simulink model "Model_Architecture"  (R2025b)
settings: Solver=VariableStepAuto  StartTime=0.0  StopTime=10.0  RelTol=1e-3
undefined symbols (not defined in the file): Selector
settings Model: Creator=dehc5901  LastModifiedBy=dehc5901

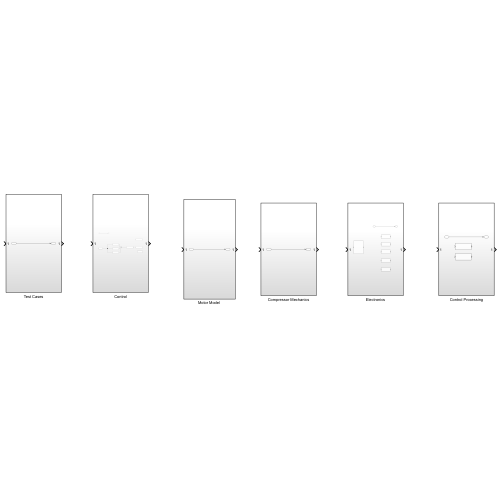
[thumbnail: Simulink's stored preview of the top-level diagram]
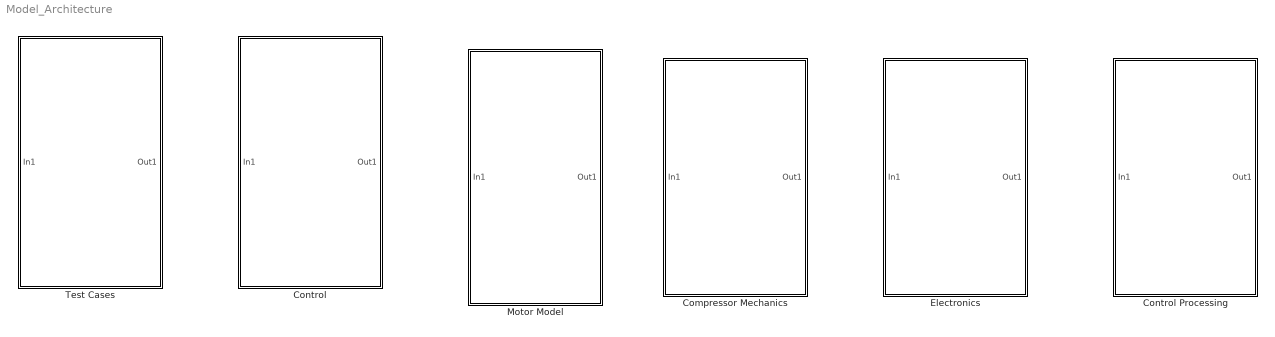
== system Model_Architecture ==
  Compressor Mechanics : Subsystem
  Control : Subsystem
  Control Processing : Subsystem
  Electronics : Subsystem
  "Motor Model " : Subsystem
  Test Cases : Subsystem

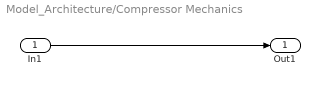
== system Model_Architecture/Compressor Mechanics ==
  In1 : Inport
  Out1 : Outport
  wires:
  In1/1 -> Out1/1

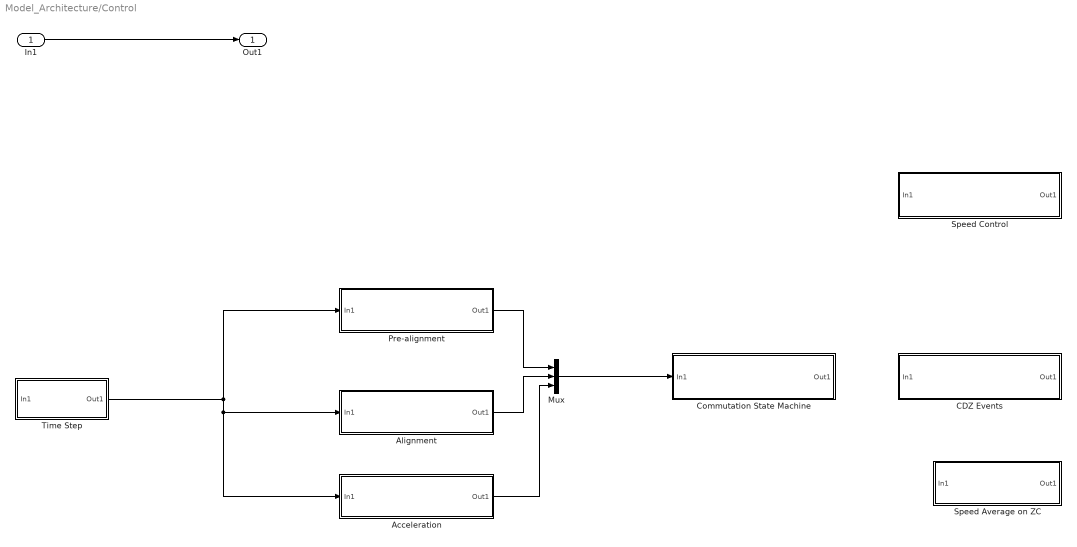
== system Model_Architecture/Control ==
  In1 : Inport
  Acceleration : Subsystem
  Alignment : Subsystem
  CDZ Events : Subsystem
  Commutation State Machine : Subsystem
  Mux : Mux  Inputs=3
  Pre-alignment : Subsystem
  Speed Average on ZC : Subsystem
  Speed Control : Subsystem
  Time Step : Subsystem
  Out1 : Outport
  wires:
  In1/1 -> Out1/1
  Mux/1 -> Commutation State Machine/1(In1)
  Pre-alignment/1(Out1) -> Mux/1
  Alignment/1(Out1) -> Mux/2
  Acceleration/1(Out1) -> Mux/3
  Time Step/1(Out1) -> Pre-alignment/1(In1), Acceleration/1(In1), Alignment/1(In1)

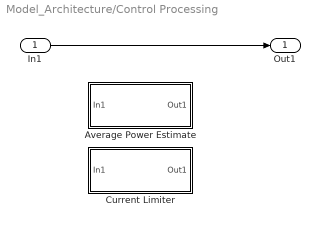
== system Model_Architecture/Control Processing ==
  In1 : Inport
  Average Power Estimate : Subsystem
  Current Limiter : Subsystem
  Out1 : Outport
  wires:
  In1/1 -> Out1/1

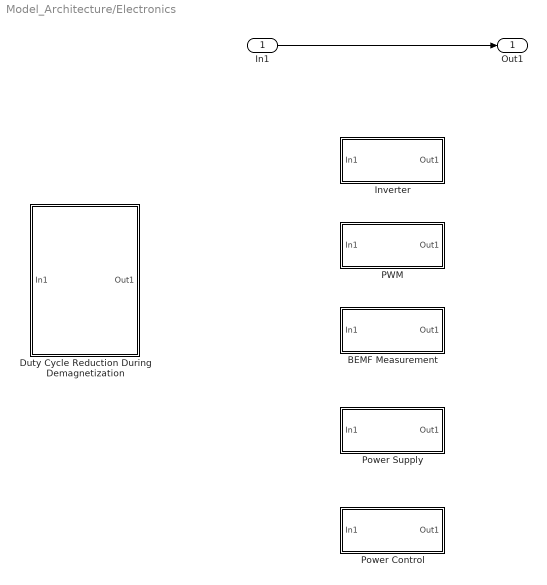
== system Model_Architecture/Electronics ==
  In1 : Inport
  BEMF Measurement : Subsystem
  Duty Cycle Reduction During Demagnetization : Subsystem
  Inverter : Subsystem
  PWM : Subsystem
  Power Control : Subsystem
  Power Supply : Subsystem
  Out1 : Outport
  wires:
  In1/1 -> Out1/1

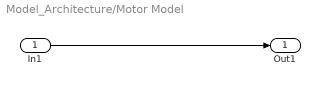
== system Model_Architecture/Motor Model  ==
  In1 : Inport
  Out1 : Outport
  wires:
  In1/1 -> Out1/1

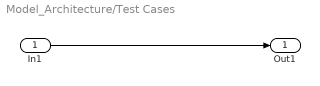
== system Model_Architecture/Test Cases ==
  In1 : Inport
  Out1 : Outport
  wires:
  In1/1 -> Out1/1

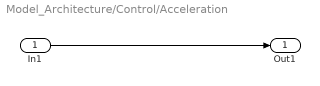
== system Model_Architecture/Control/Acceleration ==
  In1 : Inport
  Out1 : Outport
  wires:
  In1/1 -> Out1/1

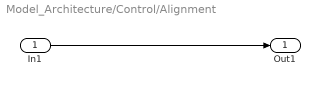
== system Model_Architecture/Control/Alignment ==
  In1 : Inport
  Out1 : Outport
  wires:
  In1/1 -> Out1/1

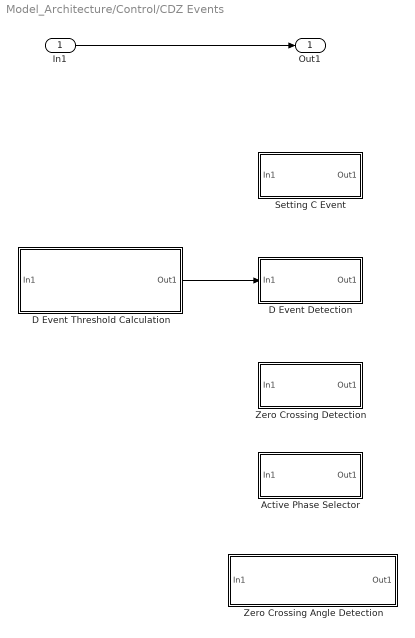
== system Model_Architecture/Control/CDZ Events ==
  In1 : Inport
  Active Phase Selector : Subsystem
  D Event Detection : Subsystem
  D Event Threshold Calculation : Subsystem
  Setting C Event : Subsystem
  "Zero Crossing Angle Detection " : Subsystem
  Zero Crossing Detection : Subsystem
  Out1 : Outport
  wires:
  In1/1 -> Out1/1
  D Event Threshold Calculation/1(Out1) -> D Event Detection/1(In1)

== system Model_Architecture/Control/Commutation State Machine ==
  In1 : Inport
  Out1 : Outport
  wires:
  In1/1 -> Out1/1

== system Model_Architecture/Control/Pre-alignment ==
  In1 : Inport
  Out1 : Outport
  wires:
  In1/1 -> Out1/1

== system Model_Architecture/Control/Speed Average on ZC ==
  In1 : Inport
  Out1 : Outport
  wires:
  In1/1 -> Out1/1

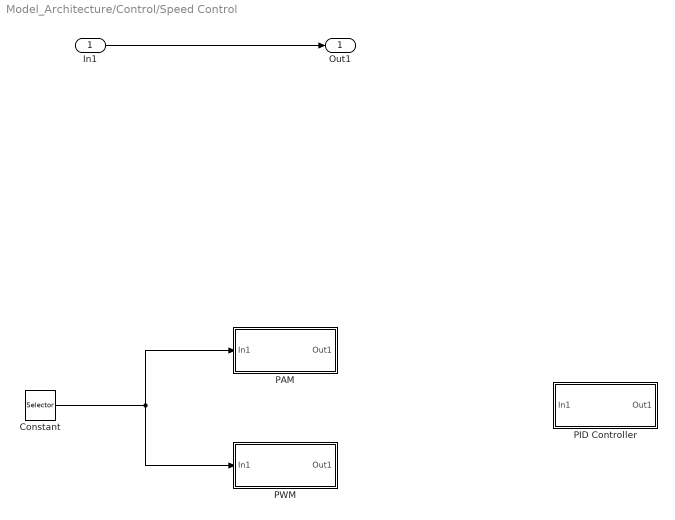
== system Model_Architecture/Control/Speed Control ==
  In1 : Inport
  Constant : Constant  Value=Selector
  PAM : Subsystem
  PID Controller : Subsystem
  PWM : Subsystem
  Out1 : Outport
  wires:
  In1/1 -> Out1/1
  Constant/1 -> PWM/1(In1), PAM/1(In1)

== system Model_Architecture/Control/Time Step ==
  In1 : Inport
  Out1 : Outport
  wires:
  In1/1 -> Out1/1

== system Model_Architecture/Control Processing/Average Power Estimate ==
  In1 : Inport
  Out1 : Outport
  wires:
  In1/1 -> Out1/1

== system Model_Architecture/Control Processing/Current Limiter ==
  In1 : Inport
  Out1 : Outport
  wires:
  In1/1 -> Out1/1

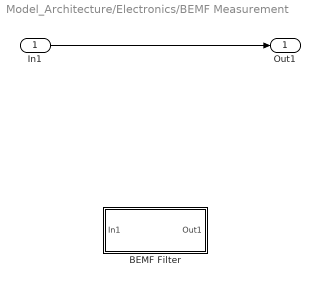
== system Model_Architecture/Electronics/BEMF Measurement ==
  In1 : Inport
  BEMF Filter : Subsystem
  Out1 : Outport
  wires:
  In1/1 -> Out1/1

== system Model_Architecture/Electronics/Duty Cycle Reduction During Demagnetization ==
  In1 : Inport
  Out1 : Outport
  wires:
  In1/1 -> Out1/1

== system Model_Architecture/Electronics/Inverter ==
  In1 : Inport
  Out1 : Outport
  wires:
  In1/1 -> Out1/1

== system Model_Architecture/Electronics/PWM ==
  In1 : Inport
  Out1 : Outport
  wires:
  In1/1 -> Out1/1

== system Model_Architecture/Electronics/Power Control ==
  In1 : Inport
  Out1 : Outport
  wires:
  In1/1 -> Out1/1

== system Model_Architecture/Electronics/Power Supply ==
  In1 : Inport
  Out1 : Outport
  wires:
  In1/1 -> Out1/1

== system Model_Architecture/Control/CDZ Events/Active Phase Selector ==
  In1 : Inport
  Out1 : Outport
  wires:
  In1/1 -> Out1/1

== system Model_Architecture/Control/CDZ Events/D Event Detection ==
  In1 : Inport
  Out1 : Outport
  wires:
  In1/1 -> Out1/1

== system Model_Architecture/Control/CDZ Events/D Event Threshold Calculation ==
  In1 : Inport
  Out1 : Outport
  wires:
  In1/1 -> Out1/1

== system Model_Architecture/Control/CDZ Events/Setting C Event ==
  In1 : Inport
  Out1 : Outport
  wires:
  In1/1 -> Out1/1

== system Model_Architecture/Control/CDZ Events/Zero Crossing Angle Detection  ==
  In1 : Inport
  Out1 : Outport
  wires:
  In1/1 -> Out1/1

== system Model_Architecture/Control/CDZ Events/Zero Crossing Detection ==
  In1 : Inport
  Out1 : Outport
  wires:
  In1/1 -> Out1/1

== system Model_Architecture/Control/Speed Control/PAM ==
  In1 : Inport
  Out1 : Outport
  wires:
  In1/1 -> Out1/1

== system Model_Architecture/Control/Speed Control/PID Controller ==
  In1 : Inport
  Out1 : Outport
  wires:
  In1/1 -> Out1/1

== system Model_Architecture/Control/Speed Control/PWM ==
  In1 : Inport
  Out1 : Outport
  wires:
  In1/1 -> Out1/1

== system Model_Architecture/Electronics/BEMF Measurement/BEMF Filter ==
  In1 : Inport
  Out1 : Outport
  wires:
  In1/1 -> Out1/1
